simulink model "V1_Fcn_Block_Model"  (R2017a)
settings: Solver=ode45  StartTime=0.0  StopTime=10.0  MaxStep=0.01  RelTol=1e-3  EnableMultiTasking=on
settings Model: Creator=ajentsch  LastModifiedBy=Ali Kerem Sacakli
settings DataIOCC: LimitDataPoints=on
settings OptimizationCC: LifeSpan=inf
settings DebuggingCC: AllowSymbolicDim=off  SFUnexpectedBacktrackingDiag=warning  SFNoUnconditionalDefaultTransitionDiag=warning  SFExecutionAtInitializationDiag=none
settings ModelReferenceCC: PropagateSignalLabelsOutOfModel=off
settings GRTTargetCC: TargetLangStandard=C89/C90 (ANSI)
settings ConfigComp: CovMetricSettings=dw  CovHtmlReporting=on  CovSaveCumulativeToWorkspaceVar=on  CovSaveSingleToWorkspaceVar=on  CovExternalEMLEnable=off

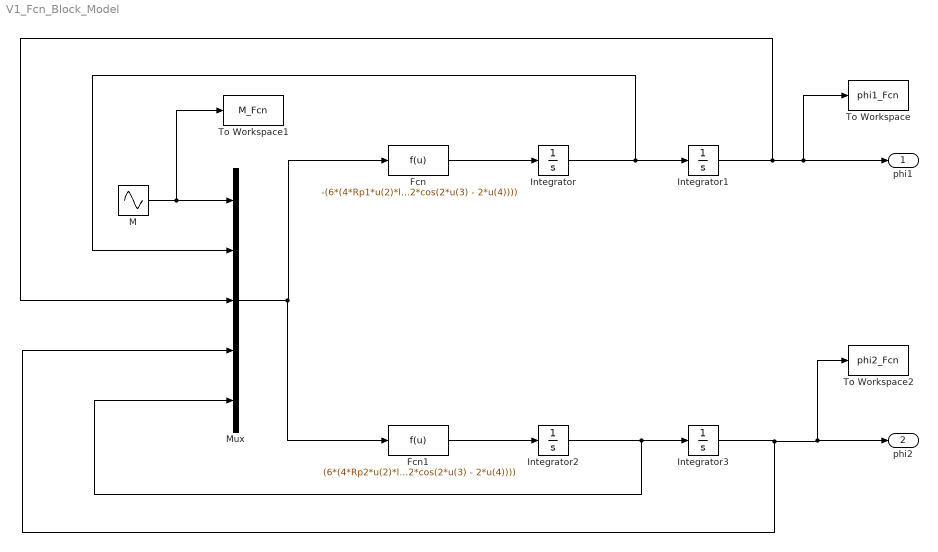
== system V1_Fcn_Block_Model ==
  Fcn : Fcn  Expr=-(6*(4*Rp1*u(2)*l2 - 4*u(1)*l2 + 6*Rp2*u(2)*l1*cos(u(3) - u(4)) - 6*Rp2*u(5)*l1*cos(u(3) - u(4)) + (3*g*l1*l2*m2*sin(u(3) - 2*u(4)))/2 + (3*u(2)^2*l1^2*l2*m2*sin(2*u(3) - 2*u(4)))/2 + 2*u(5)^2*l1*l2^2*m2*sin(u(3) - u(4)) + 2*g*l1*l2*m1*sin(u(3)) + (5*g*l1*l2*m2*sin(u(3)))/2))/(l1^2*l2*(8*m1 + 15*m2 - 9*m2*cos(2*u(3) - 2*u(4))))
  Fcn1 : Fcn  Expr=(6*(4*Rp2*u(2)*l1*m1 - 6*u(1)*l2*m2*cos(u(3) - u(4)) + 12*Rp2*u(2)*l1*m2 - 4*Rp2*u(5)*l1*m1 - 12*Rp2*u(5)*l1*m2 + 6*u(2)^2*l1^2*l2*m2^2*sin(u(3) - u(4)) - 3*g*l1*l2*m2^2*sin(u(4)) + (3*u(5)^2*l1*l2^2*m2^2*sin(2*u(3) - 2*u(4)))/2 + 3*g*l1*l2*m2^2*sin(2*u(3) - u(4)) + 6*Rp1*u(2)*l2*m2*cos(u(3) - u(4)) + 2*u(2)^2*l1^2*l2*m1*m2*sin(u(3) - u(4)) - (g*l1*l2*m1*m2*sin(u(4)))/2 + (3*g*l1*l2*m1*m2*sin(2*u(3) - u(4)))/2))/(l1*l2^2*m2*(8*m1 + 15*m2 - 9*m2*cos(2*u(3) - 2*u(4))))
  Integrator{,1..3} (4 alike) : Integrator
  M : Sin  Amplitude=0.1  SampleTime=0
  Mux : Mux  Inputs=5
  To Workspace : ToWorkspace  VariableName=phi1_Fcn  SaveFormat=Timeseries  SampleTime=-1
  To Workspace1 : ToWorkspace  VariableName=M_Fcn  SaveFormat=Timeseries  SampleTime=-1
  To Workspace2 : ToWorkspace  VariableName=phi2_Fcn  SaveFormat=Timeseries  SampleTime=-1
  phi1 : Outport
  phi2 : Outport  Port=2
  wires:
  Mux/1 -> Fcn1/1, Fcn/1
  Fcn1/1 -> Integrator2/1
  Fcn/1 -> Integrator/1
  Integrator2/1 -> Mux/5, Integrator3/1
  Integrator3/1 -> Mux/4, To Workspace2/1, phi2/1
  Integrator1/1 -> To Workspace/1, phi1/1, Mux/3
  M/1 -> To Workspace1/1, Mux/1
  Integrator/1 -> Mux/2, Integrator1/1
